simulink library "Storage_Type_12"  (R2018b)
settings: Solver=ode45  StartTime=0.0  StopTime=10.0  RelTol=1e-3  EnableMultiTasking=on
undefined symbols (not defined in the file): path_carnot
libraries: carnot x9
settings Model: Creator=bernd.hafner  LastModifiedBy=drhf
settings DataIOCC: LimitDataPoints=on  SaveFormat=Array  SignalLoggingSaveFormat=ModelDataLogs
settings OptimizationCC: ExpressionDepthLimit=2147483647  LifeSpan=inf
settings DebuggingCC: UnderspecifiedInitializationDetection=Classic  MergeDetectMultiDrivingBlocksExec=none  SolverPrmCheckMsg=warning  FcnCallInpInsideContextMsg=warning  StateNameClashWarn=warning  SFUnexpectedBacktrackingDiag=warning  SFNoUnconditionalDefaultTransitionDiag=warning  SFExecutionAtInitializationDiag=none
settings HardwareCC: ProdBitPerPointer=32  ProdBitPerSizeT=32  ProdBitPerPtrDiffT=32  ProdLargestAtomicFloat=None  ProdIntDivRoundTo=Undefined  ProdEndianess=Unspecified  ProdWordSize=32  ProdHWDeviceType=32-bit Generic
settings ModelReferenceCC: PropagateSignalLabelsOutOfModel=off
settings SFSimCC: SimUseLocalCustomCode=off
settings RTWCC: RTWUseLocalCustomCode=off
settings CodeAppCC: StateflowObjectComments=on
settings GRTTargetCC: TargetLangStandard=C89/C90 (ANSI)  GeneratePreprocessorConditionals=Disable all  CombineOutputUpdateFcns=off  GRTInterface=on
settings ConfigComp: CovMetricSettings=dw  CovHtmlReporting=on  CovSaveCumulativeToWorkspaceVar=on  CovSaveSingleToWorkspaceVar=on  CovExternalEMLEnable=off

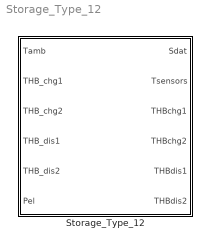
== system Storage_Type_12 ==
  Storage_Type_12 : Subsystem  mask(Buffer storage tank){t0=20, hgt=1.7684, stgtype=12, tini=[20 20 20 20 20 20 20 20 20 20], mpts=[1 2 3 4 5 6 7 8 9 10], PathName=fullfile(path_carnot('libsl'), 'Storage', 'Thermal', 'Storage_Type_12', 'parameter_set'), FileName='StorageType12_500_L.mat', userPath=off, userParam=off, uwall=1, ubot=1, utop=1, axcond=1, volume=0.5, dia=0.6, standing=standing cylinder, nodes=10, mpoints=10, Tsensor=[0.2 0.4 0.6 0.8], pipe1inlet=1, pipe1outlet=0, pipe1dia=0.05, pipe2inlet=1, pipe2outlet=0, pipe2dia=0.05, pipe3inlet=0, pipe3outlet=1, pipe3dia=0.05, pipe4inlet=0, pipe4outlet=1, pipe4dia=0.05, heater1start=0.6, heater1end=0.65}
      mask prompts: t0 "Initial temperature (vector or scalar) in °C"; hgt "Height of storage in m"; stgtype "Storage Type (0..12)"; tini "Start temperatures of nodes in °C"; mpts "Index to measured nodes"; PathName "Path"; FileName "Parameter set"; userPath "Edit path and name of parameter set"; userParam "User defined parameters"; uwall "Heat transfer coefficient to ambient [W/m²K]"; ubot "Heat transfer coefficient to ambient bottom [W/m²K]"; utop "Heat transfer coefficient to ambient top [W/m²K]"; axcond "Effective thermal conductivity [W/m/K]"; volume "Volume [m³]"; dia "Diameter [m]"; standing "Position"; nodes "Number of nodes"; mpoints "Number of node temperatures (for display)"; Tsensor "Temperature sensor position (0..1, 0 = bottom, 1 = top)"; pipe1inlet "relative height of inlet, range from 0 (= bottom) to 1 (= top)"; pipe1outlet "relative height of outlet, range from 0 (= bottom) to 1 (= top)"; pipe1dia "Diameter of pipe in m"; pipe2inlet "relative height of inlet, range from 0 (= bottom) to 1 (= top)"; pipe2outlet "relative height of outlet, range from 0 (= bottom) to 1 (= top)"; pipe2dia "Diameter of pipe in m"; pipe3inlet "relative height of inlet, range from 0 (= bottom) to 1 (= top)"; pipe3outlet "relative height of outlet, range from 0 (= bottom) to 1 (= top)"; pipe3dia "Diameter of pipe in m"; pipe4inlet "relative height of inlet, range from 0 (= bottom) to 1 (= top)"; pipe4outlet "relative height of outlet, range from 0 (= bottom) to 1 (= top)"; pipe4dia "Diameter of pipe in m"; heater1start "relative height start heating zone"; heater1end "relative height end heating zone"
      mask help:
      | Buffer storage for heating circuits. The storage model has the following components (with their typical position):
      | - one pipe connection for discharging (total height)
      | - one pipe connection for charging (total height)
      mask init:
      | [ok, param] = CarnotCallbacks_StorageConf('SetParam',stgtype,gcbh,PathName,FileName);
      mask Help: web(fullfile(path_carnot('help'),'Storage_Type_N.html'),'-helpbrowser')
      mask TypeOptions hgt: Pipe_Connection_1/hgt | Pipe_Connection_3/hgt | Pipe_Connection_2/hgt | Pipe_Connection_4/hgt
      mask TypeOptions stgtype: CreateSdat/stgtype
      mask TypeOptions tini: sfun_storageTnodes/tini
      mask TypeOptions mpts: select_T/Indices
      mask Callback userPath: [ok, param] = CarnotCallbacks_StorageConf('UserEdit',1,gcbh);
      mask Callback userParam: [ok, param] = CarnotCallbacks_StorageConf('UserEdit',1,gcbh);
      mask TypeOptions uwall: sfun_storageTnodes/uloss
      mask TypeOptions ubot: sfun_storageTnodes/ubot
      mask TypeOptions utop: sfun_storageTnodes/utop
      mask TypeOptions axcond: sfun_storageTnodes/cond
      mask TypeOptions volume: sfun_storageTnodes/volume | CreateSdat/volume
      mask TypeOptions dia: sfun_storageTnodes/dia | Pipe_Connection_1/dstg | Pipe_Connection_3/dstg | Pipe_Connection_2/dstg | Pipe_Connection_4/dstg
      mask TypeOptions standing: sfun_storageTnodes/standing
      mask TypeOptions nodes: sfun_storageTnodes/nodes | select_T/InputPortWidth | Pipe_Connection_1/nodes | Pipe_Connection_3/nodes | Pipe_Connection_2/nodes | Pipe_Connection_4/nodes
      mask TypeOptions Tsensor: T_Sensor_Surface/pos
      mask TypeOptions pipe1inlet: Pipe_Connection_1/h_in
      mask TypeOptions pipe1outlet: Pipe_Connection_1/h_out
      mask TypeOptions pipe1dia: Pipe_Connection_1/dpipe
      mask TypeOptions pipe2inlet: Pipe_Connection_2/h_in
      mask TypeOptions pipe2outlet: Pipe_Connection_2/h_out
      mask TypeOptions pipe2dia: Pipe_Connection_2/dpipe
      mask TypeOptions pipe3inlet: Pipe_Connection_3/h_in
      mask TypeOptions pipe3outlet: Pipe_Connection_3/h_out
      mask TypeOptions pipe3dia: Pipe_Connection_3/dpipe
      mask TypeOptions pipe4inlet: Pipe_Connection_4/h_in
      mask TypeOptions pipe4outlet: Pipe_Connection_4/h_out
      mask TypeOptions pipe4dia: Pipe_Connection_4/dpipe
      mask TypeOptions heater1start: Electric_Heating_1/hin
      mask TypeOptions heater1end: Electric_Heating_1/hout
      mask DialogControl Container14 Prompt: Infos
      mask DialogControl ParameterGroupVar Prompt: Picking a parameter set
      mask DialogControl Control3 Prompt: Carnot public data
      mask DialogControl Control3 Callback: [ok, file] = CarnotCallbacks_StorageConf('GetFilename',12,gcbh,'public');
      mask DialogControl Control4 Prompt: Carnot internal data
      mask DialogControl Control4 Callback: [ok, file] = CarnotCallbacks_StorageConf('GetFilename',12,gcbh,'internal');
      mask DialogControl Control2 Prompt: Selected path
      mask DialogControl Control2 Callback: [ok, file] = CarnotCallbacks_StorageConf('GetFilename',12,gcbh,'selected');
      mask DialogControl Container4 Prompt: Parameter values
      mask DialogControl Container6 Prompt: Storage
      mask DialogControl Container8 Prompt: Connections
      mask DialogControl Container9 Prompt: Charging pipe 1
      mask DialogControl Container18 Prompt: Charging pipe 2
      mask DialogControl Container12 Prompt: Discharging pipe 1
      mask DialogControl Container19 Prompt: Discharging pipe 2
      mask DialogControl Container13 Prompt: Electric Heating
      mask DialogControl Container15 Prompt: Heater 1
      mask DialogControl Control6 Prompt: Save in Carnot internal data
      mask DialogControl Control6 Callback: [ok, param] = CarnotCallbacks_StorageConf('SaveFilename',12,gcbh,'internal','STG');
      mask DialogControl Control5 Prompt: Save in selected path
      mask DialogControl Control5 Callback: [ok, param] = CarnotCallbacks_StorageConf('SaveFilename',12,gcbh,'selected','STG');
      mask Display:
      | % user defined picture file
      | namestr = ['Storage_Type_', num2str(get_param(gcb,'stgtype'))];
      | picfile = fullfile(path_carnot('intlibsl'), 'Storage','Thermal', ...
      |     namestr,'parameter_set', [namestr, '.jpg']);
      | 
      | % show internal picture if defined
      | pic = false;
      | if  ~BlockIsInCarnotLibrary       % if not located in library
      |     if exist(picfile, 'file')
      |         image(imread(picfile), [0.25, 0, 0.45, 1])
      |         set_param(gcb, 'BackgroundColor', 'White')
      |         pic = true;
      |     end
      | end
      | 
      | % show public picture
      | if ~pic
      |     set_param(gcb, 'BackgroundColor', 'Red')
      |     plot([40,40,45,55,60,60,55,45,40]/100,[84,36,30,30,36,84,90,90,84]/100, ...
      |         [40,35]/100,[77,77]/100,...
      |         [40,35]/100,[85,85]/100,...
      |         [64,60]/100,[77,77]/100,...
      |         [64,60]/100,[85,85]/100,...
      |         [40,35]/100,[42,42]/100, ...
      |         [40,35]/100,[35,35]/100, ...
      |         [64,60]/100,[42,42]/100,...
      |         [64,60]/100,[35,35]/100,...
      |         [40,55,55,40]/100,[72,72,70.5,70.5]/100,...
      |         [40,38,38,40]/100,[73,73,69,69]/100)
      | end

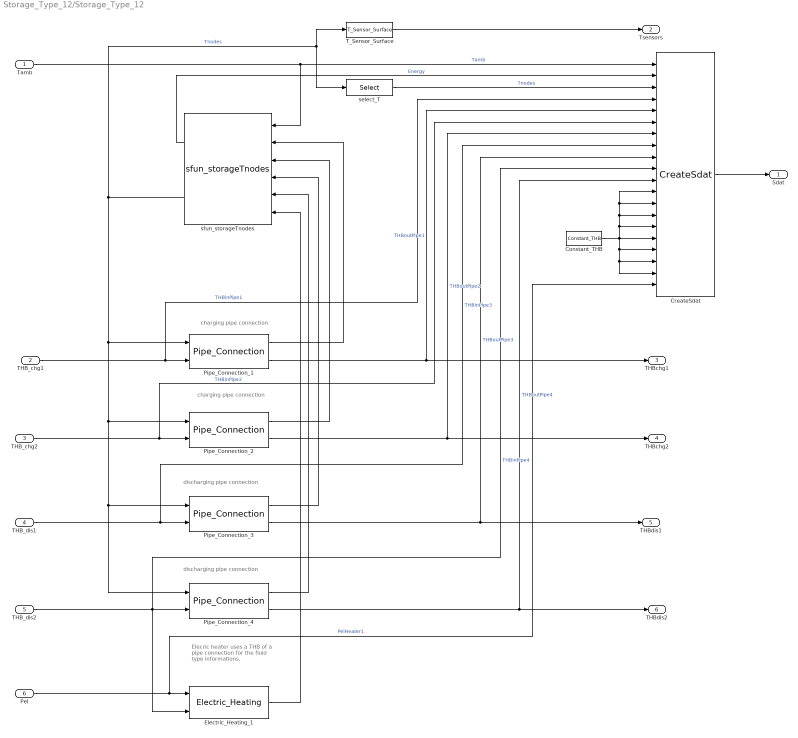
== system Storage_Type_12/Storage_Type_12 ==
  note: discharging pipe connection
  note: charging pipe connection
  note: discharging pipe connection
  note: charging pipe connection
  note: Elecric heater uses a THB of
      | a pipe connection for the fluid
      | type informations.
  Tamb : Inport
  THB_chg1 : Inport  Port=2
  THB_chg2 : Inport  Port=3
  THB_dis1 : Inport  Port=4
  THB_dis2 : Inport  Port=5
  Pel : Inport  Port=6
  Constant_THB : carnot/Source/Simple/Constant_THB  t=20  mdot=0  p=1e5  mID=No Pressure Drop  fluid=Water  mix=0  mix2=0  mix3=0  dia=0.02  hgt=0
      settings: SourceProductName=Carnot
  CreateSdat : carnot/Basic/Thermal_Models/CreateSdat  volume=volume  stgtype=stgtype
      settings: SourceProductName=Carnot
  Electric_Heating_1 : carnot/Storage/Thermal/Storage_Ports/Electric_Heating  hin=heater1start  hout=heater1end  nodes=nodes
      settings: SourceProductName=Carnot
  Pipe_Connection_1 : carnot/Storage/Thermal/Storage_Ports/Pipe_Connection  h_in=pipe1inlet  h_out=pipe1outlet  hgt=hgt  dpipe=pipe1dia  dstg=dia  height=-1.7684  nodes=nodes
      settings: SourceProductName=Carnot
  Pipe_Connection_2 : carnot/Storage/Thermal/Storage_Ports/Pipe_Connection  h_in=pipe2inlet  h_out=pipe2outlet  hgt=hgt  dpipe=pipe2dia  dstg=dia  height=-1.7684  nodes=nodes
      settings: SourceProductName=Carnot
  Pipe_Connection_3 : carnot/Storage/Thermal/Storage_Ports/Pipe_Connection  h_in=pipe3inlet  h_out=pipe3outlet  hgt=hgt  dpipe=pipe3dia  dstg=dia  height=1.7684  nodes=nodes
      settings: SourceProductName=Carnot
  Pipe_Connection_4 : carnot/Storage/Thermal/Storage_Ports/Pipe_Connection  h_in=pipe4inlet  h_out=pipe4outlet  hgt=hgt  dpipe=pipe4dia  dstg=dia  height=1.7684  nodes=nodes
      settings: SourceProductName=Carnot
  T_Sensor_Surface : carnot/Control/T_Sensor_Surface  pos=Tsensor  tdel=10  t0=mean(tini)
      settings: SourceProductName=Carnot
  select_T : Selector  InputPortWidth=nodes  IndexOptions=Index vector (dialog)  Indices=[1 2 3 4 5 6 7 8 9 10]  OutputSizes=1
  sfun_storageTnodes : carnot/Basic/Thermal_Models/sfun_storageTnodes  uloss=uwall  ubot=ubot  utop=utop  cond=axcond  volume=volume  dia=dia  standing=standing cylinder  tini=tini  nodes=nodes  nconnect=5  elimthermocline=2  condinvtc=1e5
      settings: SourceProductName=Carnot
  Sdat : Outport
  Tsensors : Outport  Port=2
  THBchg1 : Outport  Port=3
  THBchg2 : Outport  Port=4
  THBdis1 : Outport  Port=5
  THBdis2 : Outport  Port=6
  wires:
  Constant_THB/1 -> CreateSdat/16, CreateSdat/12, CreateSdat/13, CreateSdat/14, CreateSdat/15, CreateSdat/19, CreateSdat/18, CreateSdat/17
  T_Sensor_Surface/1 -> Tsensors/1
  Pipe_Connection_1/1 -> sfun_storageTnodes/2
  Pipe_Connection_1/2 -> THBchg1/1, CreateSdat/5  "THBoutPipe1"
  THB_chg1/1 -> Pipe_Connection_1/2, CreateSdat/4  "THBinPipe1"
  select_T/1 -> CreateSdat/3  "Tnodes"
  Tamb/1 -> CreateSdat/1, sfun_storageTnodes/1  "Tamb"
  Pipe_Connection_3/1 -> sfun_storageTnodes/4
  Pipe_Connection_3/2 -> THBdis1/1, CreateSdat/9  "THBoutPipe3"
  sfun_storageTnodes/1 -> CreateSdat/2  "Energy"
  Pel/1 -> Electric_Heating_1/1, CreateSdat/20  "PelHeater1"
  THB_dis1/1 -> Pipe_Connection_3/2, CreateSdat/8  "THBinPipe3"
  Electric_Heating_1/1 -> sfun_storageTnodes/6
  THB_dis2/1 -> Electric_Heating_1/2, Pipe_Connection_4/2, CreateSdat/10  "THBinPipe4"
  Pipe_Connection_4/2 -> THBdis2/1, CreateSdat/11  "THBoutPipe4"
  Pipe_Connection_4/1 -> sfun_storageTnodes/5
  sfun_storageTnodes/2 -> Pipe_Connection_1/1, Pipe_Connection_4/1, Pipe_Connection_3/1, Pipe_Connection_2/1, select_T/1, T_Sensor_Surface/1  "Tnodes"
  THB_chg2/1 -> Pipe_Connection_2/2, CreateSdat/6  "THBinPipe2"
  Pipe_Connection_2/2 -> THBchg2/1, CreateSdat/7  "THBoutPipe2"
  Pipe_Connection_2/1 -> sfun_storageTnodes/3
  CreateSdat/1 -> Sdat/1
